simulink model "narmaL2"  (R2016b)
settings: Solver=ode45  StartTime=0.0  StopTime=600  RelTol=1e-3  AbsTol=1e-8  EnableMultiTasking=on
values from neighbouring files (symbols this model uses):
  Ar = 6*25.4    (= 152.4)    [param2NL.m]
  hmax = 16    [param2NL.m]
  k12 = 38    [param2NL.m]
  k2 = 11.5    [param2NL.m]
  qmax = 90    [param2NL.m]
  qmin = 0    [param2NL.m]
libraries: neural x1
settings Model: Creator=Adolfo  LastModifiedBy=adolfobs
settings DataIOCC: LimitDataPoints=on  SaveFormat=Array  SignalLoggingSaveFormat=ModelDataLogs
settings OptimizationCC: ExpressionDepthLimit=2147483647  InitFltsAndDblsToZero=on  LifeSpan=inf
settings DebuggingCC: SaveWithParameterizedLinksMsg=none  UnderspecifiedInitializationDetection=Classic  MergeDetectMultiDrivingBlocksExec=none  SignalResolutionControl=TryResolveAllWithWarning  SolverPrmCheckMsg=warning  MultiTaskDSMMsg=warning  MultiTaskCondExecSysMsg=none  FcnCallInpInsideContextMsg=warning  StateNameClashWarn=warning  StrictBusMsg=None  SFUnexpectedBacktrackingDiag=warning  SFNoUnconditionalDefaultTransitionDiag=warning  SFExecutionAtInitializationDiag=none
settings HardwareCC: ProdBitPerPointer=32  ProdBitPerSizeT=32  ProdBitPerPtrDiffT=32  ProdLargestAtomicFloat=None  ProdIntDivRoundTo=Undefined  ProdEndianess=Unspecified  ProdWordSize=32  ProdHWDeviceType=32-bit Generic
settings ModelReferenceCC: PropagateSignalLabelsOutOfModel=off
settings GRTTargetCC: TargetFcnLib=ansi_tfl_tmw.mat  TargetLangStandard=C89/C90 (ANSI)  GeneratePreprocessorConditionals=Disable all  CombineOutputUpdateFcns=off  GRTInterface=on
settings ConfigComp: CovMetricSettings=dw  CovHtmlReporting=on  CovSaveCumulativeToWorkspaceVar=on  CovSaveSingleToWorkspaceVar=on  CovExternalEMLEnable=off

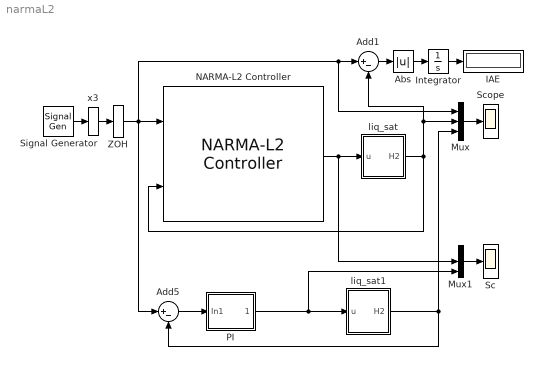
== system narmaL2 ==
  Abs : Abs
  Add1 : Sum  Inputs=|+-
  Add5 : Sum  Inputs=|+-
  IAE : Display
  Integrator : Integrator
  Mux : Mux  Inputs=3
  Mux1 : Mux  Inputs=3
  NARMA-L2 Controller : neural/Control Systems/NARMA-L2 Controller  Normalize=[]  IW1_1=[]  IW3_2=[]  IW5_3=[]  LW2_1=[]  LW4_3=[]  LW5_4=[]  LW6_5=[]  LW6_2=[]  B1=[]  B2=[]  B3=[]  B4=[]  Limit_output=[]  min_output=[]  max_output=[]  Use_Previous_Weights=[]  Ts=[]  S1=[]  Ni=[]  Nj=[]  sim_file=0  trainfun=trainlm  Use_validation=[]  Use_Testing=[]  max_i=[]  min_i=[]  max_i_int=[]  min_i_int=[]  sam_training=[]  epochs=[]  minp=[]  maxp=[]  mint=[]  maxt=[]
  PI : Subsystem
  Sc : Scope
  Scope : Scope
  Signal Generator : SignalGenerator  WaveForm=square  Amplitude=-12/300  Frequency=1/600
  ZOH : ZeroOrderHold  SampleTime=100
  liq_sat : Subsystem
  liq_sat1 : Subsystem
  x3 : Integrator
  wires:
  Mux/1 -> Scope/1
  NARMA-L2 Controller/1 -> Mux1/2, liq_sat/1(u)
  PI/1(Out1) -> Mux1/3, liq_sat1/1(u)
  Add5/1 -> PI/1(In1)
  Mux1/1 -> Sc/1
  liq_sat1/1(H2) -> Add5/2, Mux/3
  liq_sat/1(H2) -> Mux/2, Add1/2, NARMA-L2 Controller/2
  Signal Generator/1 -> x3/1
  x3/1 -> ZOH/1
  ZOH/1 -> Add5/1, Mux/1, Add1/1, NARMA-L2 Controller/1
  Add1/1 -> Abs/1
  Abs/1 -> Integrator/1
  Integrator/1 -> IAE/1

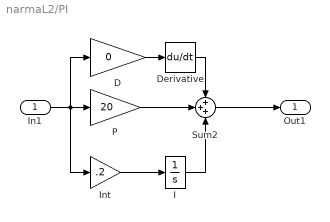
== system narmaL2/PI ==
  In1 : Inport
  D : Gain  Gain=0
  Derivative : Derivative
  I : Integrator
  Int : Gain  Gain=.2
  P : Gain  Gain=20
  Sum2 : Sum  Inputs=+++
  Out1 : Outport
  wires:
  In1/1 -> P/1, Int/1, D/1
  P/1 -> Sum2/2
  I/1 -> Sum2/3
  Sum2/1 -> Out1/1
  Int/1 -> I/1
  D/1 -> Derivative/1
  Derivative/1 -> Sum2/1

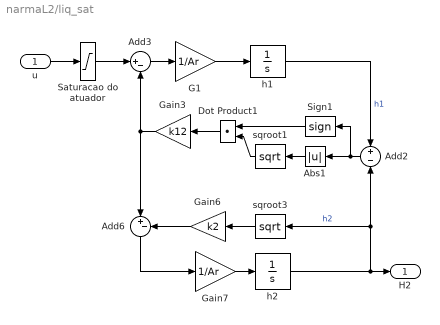
== system narmaL2/liq_sat ==
  u : Inport
  Abs1 : Abs
  Add2 : Sum  Inputs=+-
  Add3 : Sum  Inputs=|+-
  Add6 : Sum  Inputs=|+-
  Dot Product1 : DotProduct  InputSameDT=on  OutDataTypeStr=Inherit: Inherit via internal rule
  G1 : Gain  Gain=1/Ar
  Gain3 : Gain  Gain=k12
  Gain6 : Gain  Gain=k2
  Gain7 : Gain  Gain=1/Ar
  Saturacao do atuador : Saturate  UpperLimit=qmax  LowerLimit=qmin
  Sign1 : Signum
  h1 : Integrator  LimitOutput=on  UpperSaturationLimit=hmax  LowerSaturationLimit=0
  h2 : Integrator  LimitOutput=on  UpperSaturationLimit=hmax  LowerSaturationLimit=0
  sqroot1 : Math  Operator=sqrt  SaturateOnIntegerOverflow=on
  sqroot3 : Math  Operator=sqrt  SaturateOnIntegerOverflow=on
  H2 : Outport
  wires:
  h1/1 -> Add2/1  "h1"
  h2/1 -> Add2/2, sqroot3/1, H2/1  "h2"
  Saturacao do atuador/1 -> Add3/1
  Add6/1 -> Gain7/1
  Gain6/1 -> Add6/2
  Gain7/1 -> h2/1
  sqroot3/1 -> Gain6/1
  G1/1 -> h1/1
  Gain3/1 -> Add6/1, Add3/2
  Add3/1 -> G1/1
  Dot Product1/1 -> Gain3/1
  sqroot1/1 -> Dot Product1/2
  Sign1/1 -> Dot Product1/1
  Abs1/1 -> sqroot1/1
  Add2/1 -> Abs1/1, Sign1/1
  u/1 -> Saturacao do atuador/1

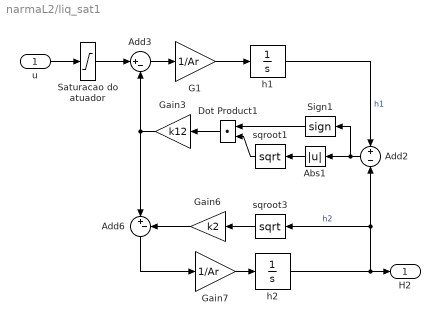
== system narmaL2/liq_sat1 ==
  u : Inport
  Abs1 : Abs
  Add2 : Sum  Inputs=+-
  Add3 : Sum  Inputs=|+-
  Add6 : Sum  Inputs=|+-
  Dot Product1 : DotProduct  InputSameDT=on  OutDataTypeStr=Inherit: Inherit via internal rule
  G1 : Gain  Gain=1/Ar
  Gain3 : Gain  Gain=k12
  Gain6 : Gain  Gain=k2
  Gain7 : Gain  Gain=1/Ar
  Saturacao do atuador : Saturate  UpperLimit=qmax  LowerLimit=qmin
  Sign1 : Signum
  h1 : Integrator  LimitOutput=on  UpperSaturationLimit=hmax  LowerSaturationLimit=0
  h2 : Integrator  LimitOutput=on  UpperSaturationLimit=hmax  LowerSaturationLimit=0
  sqroot1 : Math  Operator=sqrt  SaturateOnIntegerOverflow=on
  sqroot3 : Math  Operator=sqrt  SaturateOnIntegerOverflow=on
  H2 : Outport
  wires:
  h1/1 -> Add2/1  "h1"
  h2/1 -> Add2/2, sqroot3/1, H2/1  "h2"
  Saturacao do atuador/1 -> Add3/1
  Add6/1 -> Gain7/1
  Gain6/1 -> Add6/2
  Gain7/1 -> h2/1
  sqroot3/1 -> Gain6/1
  G1/1 -> h1/1
  Gain3/1 -> Add6/1, Add3/2
  Add3/1 -> G1/1
  Dot Product1/1 -> Gain3/1
  sqroot1/1 -> Dot Product1/2
  Sign1/1 -> Dot Product1/1
  Abs1/1 -> sqroot1/1
  Add2/1 -> Abs1/1, Sign1/1
  u/1 -> Saturacao do atuador/1
